simulink model "sampleModel1805"  (R2023a)
settings: Solver=VariableStepAuto  StartTime=0.0  StopTime=10.0  RelTol=1e-3
libraries: hdlsllib x3
settings Model: Creator=user1  LastModifiedBy=user1

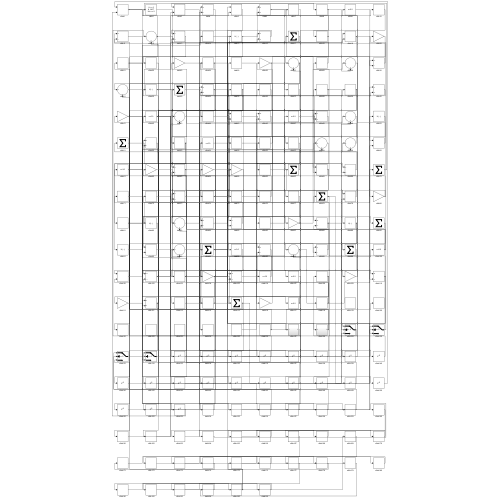
[thumbnail: Simulink's stored preview of the top-level diagram]
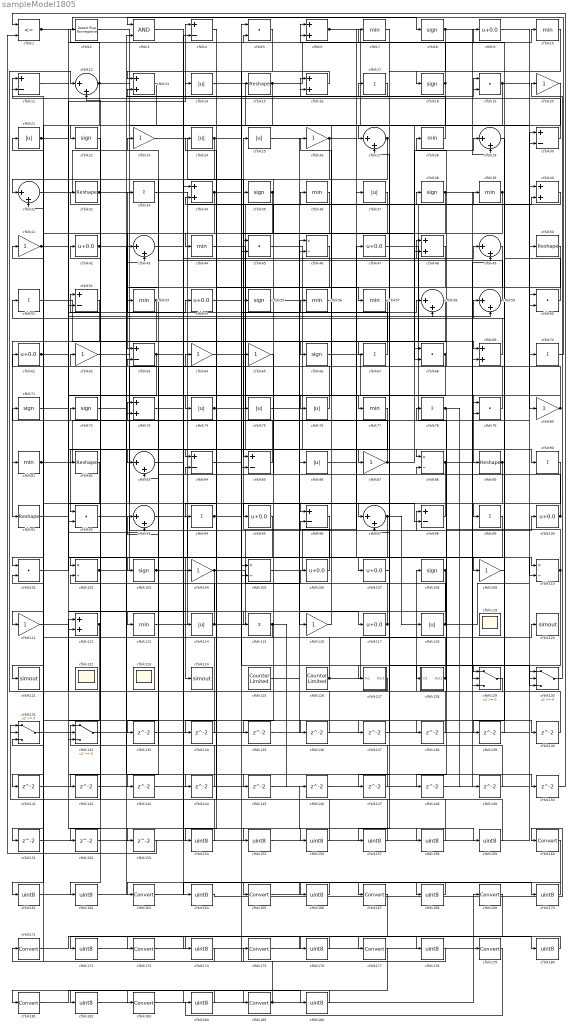
== system sampleModel1805 ==
  cfblk1 : RelationalOperator  Operator=<=  OutDataTypeStr=boolean  InputSameDT=off
  cfblk{7,10,28,36,39,44,53,56..57,77,81,113} (12 alike) : MinMax
  cfblk{9,42,47,54,61,95,100,106..107,117} (10 alike) : Bias  Bias=0.0  SaturateOnIntegerOverflow=off
  cfblk{5,19,45,60,68,79,92,101} (8 alike) : DotProduct  OutDataTypeStr=Inherit: Inherit via internal rule
  cfblk{46,88,102,105,110} (5 alike) : Product  Inputs=*/  RndMeth=Zero  SaturateOnIntegerOverflow=on
  cfblk{8,18,22,35,38,55,66,71..72,103,108} (11 alike) : Signum
  cfblk{20,23,26,41,62,64..65,80,87,104,109,111,116} (13 alike) : Gain
  cfblk{4,11,30,52,63,84..85,96,98} (9 alike) : Sum  Inputs=+-
  cfblk{6,13,16,34,40,48,69,73,112} (9 alike) : Sum
  cfblk{14,21,24..25,37,74..76,86,114,118} (11 alike) : Abs  SaturateOnIntegerOverflow=off
  cfblk{17,33,51,67,70,78,90,94,99,115} (10 alike) : Sum  Inputs=+
  cfblk119 : Scope
      settings: Floating=on
  cfblk{12,27,29,31,43,49,58..59,83,93,97} (11 alike) : Sum  Inputs=|++
  cfblk120 : ToWorkspace  VariableName=simout  SaveFormat=Timeseries  SampleTime=-1
  cfblk121 : ToWorkspace  VariableName=simout  SaveFormat=Timeseries  SampleTime=-1
  cfblk122 : Scope
      settings: Floating=on
  cfblk123 : Scope
      settings: Floating=on
  cfblk124 : ToWorkspace  VariableName=simout  SaveFormat=Timeseries  SampleTime=-1
  cfblk125 : hdlsllib/Sources/Counter Limited  uplimit=7  tsamp=-1
  cfblk126 : hdlsllib/Sources/Counter Limited  uplimit=7  tsamp=-1
  cfblk127 : Subsystem
      settings: LibrarySourceBlock=|
      | hdlsllib/Ports &
      | Subsystems/Subsystem
  cfblk128 : Subsystem
      settings: LibrarySourceBlock=|
      | hdlsllib/Ports &
      | Subsystems/Subsystem
  cfblk{129..132} (4 alike) : Switch  SaturateOnIntegerOverflow=off  InputSameDT=off
  cfblk{133..153} (21 alike) : Delay  SampleTime=1
  cfblk{15,32,50,82,89,91} (6 alike) : Reshape
  cfblk{154..159,161..162,164,166,168,170,172,174,176,178,180,182,184,186} (20 alike) : DataTypeConversion  OutDataTypeStr=uint8  SaturateOnIntegerOverflow=off  RndMeth=Floor
  cfblk{160,163,165,167,169,171,173,175,177,179,181,183,185} (13 alike) : DataTypeConversion  SaturateOnIntegerOverflow=off  RndMeth=Floor
  cfblk2 : hdlsllib/Logic and Bit Operations/Detect Rise Nonnegative  vinit=0  OutDataTypeStr=boolean
  cfblk3 : Logic  AllPortsSameDT=off  OutDataTypeStr=boolean
  wires:
  cfblk98/1 -> cfblk62/1
  cfblk78/1 -> cfblk148/1, cfblk149/1
  cfblk113/1 -> cfblk36/1
  cfblk56/1 -> cfblk31/1
  cfblk110/1 -> cfblk39/1, cfblk129/1, cfblk147/1
  cfblk18/1 -> cfblk27/1, cfblk6/2
  cfblk89/1 -> cfblk99/1, cfblk135/1
  cfblk45/1 -> cfblk90/1
  cfblk64/1 -> cfblk77/1
  cfblk93/1 -> cfblk109/1
  cfblk106/1 -> cfblk25/1
  cfblk32/1 -> cfblk96/1, cfblk7/1
  cfblk92/1 -> cfblk96/2
  cfblk23/1 -> cfblk85/1
  cfblk66/1 -> cfblk89/1
  cfblk115/1 -> cfblk31/2, cfblk146/1
  cfblk105/1 -> cfblk47/1
  cfblk30/1 -> cfblk11/1
  cfblk96/1 -> cfblk124/1
  cfblk74/1 -> cfblk38/1, cfblk127/1(In1)
  cfblk2/1 -> cfblk57/1
  cfblk4/1 -> cfblk74/1
  cfblk127/1(Out1) -> cfblk12/1
  cfblk70/1 -> cfblk3/1
  cfblk52/1 -> cfblk91/1
  cfblk84/1 -> cfblk78/1
  cfblk53/1 -> cfblk81/1, cfblk73/2
  cfblk117/1 -> cfblk56/1, cfblk113/1
  cfblk20/1 -> cfblk76/1
  cfblk132/1 -> cfblk46/1
  cfblk49/1 -> cfblk66/1
  cfblk100/1 -> cfblk35/1, cfblk71/1
  cfblk82/1 -> cfblk111/1
  cfblk44/1 -> cfblk116/1
  cfblk35/1 -> cfblk63/1, cfblk162/1
  cfblk12/1 -> cfblk30/2, cfblk2/1, cfblk151/1
  cfblk34/1 -> cfblk102/1, cfblk48/2
  cfblk125/1 -> cfblk46/2
  cfblk116/1 -> cfblk26/1
  cfblk51/1 -> cfblk86/1
  cfblk19/1 -> cfblk60/1, cfblk45/2
  cfblk37/1 -> cfblk55/1
  cfblk90/1 -> cfblk97/1
  cfblk13/1 -> cfblk22/1
  cfblk8/1 -> cfblk29/2, cfblk157/1
  cfblk67/1 -> cfblk33/1
  cfblk80/1 -> cfblk79/1, cfblk11/2
  cfblk108/1 -> cfblk115/1, cfblk143/1
  cfblk107/1 -> cfblk132/1
  cfblk114/1 -> cfblk100/1, cfblk83/2
  cfblk77/1 -> cfblk92/1
  cfblk14/1 -> cfblk37/1
  cfblk126/1 -> cfblk21/1, cfblk120/1
  cfblk58/1 -> cfblk121/1
  cfblk55/1 -> cfblk69/1
  cfblk76/1 -> cfblk65/1
  cfblk75/1 -> cfblk117/1
  cfblk25/1 -> cfblk67/1
  cfblk27/1 -> cfblk53/1, cfblk44/1
  cfblk15/1 -> cfblk10/1, cfblk52/2
  cfblk16/1 -> cfblk13/1
  cfblk31/1 -> cfblk3/2
  cfblk9/1 -> cfblk80/1
  cfblk103/1 -> cfblk98/1, cfblk16/1
  cfblk39/1 -> cfblk92/2, cfblk142/1
  cfblk85/1 -> cfblk32/1
  cfblk62/1 -> cfblk87/1
  cfblk21/1 -> cfblk75/1, cfblk107/1
  cfblk6/1 -> cfblk68/1, cfblk58/2
  cfblk112/1 -> cfblk72/1, cfblk161/1
  cfblk101/1 -> cfblk54/1
  cfblk86/1 -> cfblk48/1
  cfblk60/1 -> cfblk6/1
  cfblk10/1 -> cfblk18/1
  cfblk130/1 -> cfblk20/1
  cfblk79/1 -> cfblk28/1
  cfblk129/1 -> cfblk108/1
  cfblk17/1 -> cfblk13/2
  cfblk128/1(Out1) -> cfblk52/1, cfblk41/1
  cfblk1/1 -> cfblk8/1, cfblk5/2, cfblk159/1
  cfblk81/1 -> cfblk60/2, cfblk114/1
  cfblk97/1 -> cfblk132/2, cfblk118/1
  cfblk33/1 -> cfblk40/2
  cfblk59/1 -> cfblk23/1
  cfblk48/1 -> cfblk94/1
  cfblk68/1 -> cfblk83/1, cfblk133/1
  cfblk11/1 -> cfblk84/1
  cfblk118/1 -> cfblk12/2, cfblk64/1, cfblk70/1
  cfblk95/1 -> cfblk104/1
  cfblk5/1 -> cfblk85/2
  cfblk102/1 -> cfblk15/1, cfblk19/2
  cfblk38/1 -> cfblk110/1, cfblk141/1
  cfblk57/1 -> cfblk82/1
  cfblk42/1 -> cfblk68/2, cfblk144/1, cfblk145/1
  cfblk28/1 -> cfblk4/1
  cfblk65/1 -> cfblk95/1
  cfblk26/1 -> cfblk45/1, cfblk110/2
  cfblk7/1 -> cfblk97/2
  cfblk61/1 -> cfblk59/2, cfblk14/1
  cfblk104/1 -> cfblk106/1, cfblk132/3, cfblk58/1, cfblk17/1
  cfblk36/1 -> cfblk103/1
  cfblk109/1 -> cfblk9/1
  cfblk46/1 -> cfblk105/2
  cfblk54/1 -> cfblk88/1
  cfblk91/1 -> cfblk98/2
  cfblk69/1 -> cfblk51/1
  cfblk87/1 -> cfblk73/1, cfblk29/1
  cfblk83/1 -> cfblk49/1
  cfblk88/1 -> cfblk130/3, cfblk84/2
  cfblk40/1 -> cfblk34/2
  cfblk41/1 -> cfblk93/2, cfblk140/1
  cfblk24/1 -> cfblk101/1, cfblk19/1
  cfblk63/1 -> cfblk112/2, cfblk136/1
  cfblk94/1 -> cfblk128/1(In1), cfblk129/2, cfblk16/2
  cfblk47/1 -> cfblk69/2
  cfblk133/1 -> cfblk130/2
  cfblk99/1 -> cfblk134/1
  cfblk134/1 -> cfblk34/1
  cfblk135/1 -> cfblk49/2
  cfblk136/1 -> cfblk101/2
  cfblk72/1 -> cfblk137/1
  cfblk137/1 -> cfblk27/2
  cfblk73/1 -> cfblk138/1
  cfblk138/1 -> cfblk112/1
  cfblk29/1 -> cfblk139/1
  cfblk139/1 -> cfblk59/1
  cfblk140/1 -> cfblk88/2
  cfblk141/1 -> cfblk105/1
  cfblk142/1 -> cfblk79/2
  cfblk143/1 -> cfblk130/1
  cfblk144/1 -> cfblk63/2
  cfblk146/1 -> cfblk129/3
  cfblk147/1 -> cfblk93/1
  cfblk148/1 -> cfblk30/1
  cfblk149/1 -> cfblk102/2
  cfblk111/1 -> cfblk150/1
  cfblk150/1 -> cfblk1/1
  cfblk151/1 -> cfblk4/2
  cfblk22/1 -> cfblk152/1
  cfblk152/1 -> cfblk40/1
  cfblk71/1 -> cfblk153/1
  cfblk153/1 -> cfblk1/2
  cfblk50/1 -> cfblk154/1
  cfblk154/1 -> cfblk42/1
  cfblk3/1 -> cfblk155/1
  cfblk155/1 -> cfblk50/1
  cfblk131/1 -> cfblk156/1
  cfblk156/1 -> cfblk24/1
  cfblk157/1 -> cfblk131/1
  cfblk145/1 -> cfblk158/1
  cfblk158/1 -> cfblk131/2
  cfblk159/1 -> cfblk131/3
  cfblk161/1 -> cfblk43/1
  cfblk162/1 -> cfblk43/2
  cfblk43/1 -> cfblk164/1
  cfblk164/1 -> cfblk160/1
  cfblk160/1 -> cfblk166/1
  cfblk166/1 -> cfblk163/1
  cfblk163/1 -> cfblk168/1
  cfblk168/1 -> cfblk165/1
  cfblk165/1 -> cfblk170/1
  cfblk170/1 -> cfblk167/1
  cfblk167/1 -> cfblk172/1
  cfblk172/1 -> cfblk169/1
  cfblk169/1 -> cfblk174/1
  cfblk174/1 -> cfblk171/1
  cfblk171/1 -> cfblk176/1
  cfblk176/1 -> cfblk173/1
  cfblk173/1 -> cfblk178/1
  cfblk178/1 -> cfblk175/1
  cfblk175/1 -> cfblk180/1
  cfblk180/1 -> cfblk177/1
  cfblk177/1 -> cfblk182/1
  cfblk182/1 -> cfblk179/1
  cfblk183/1 -> cfblk185/1
  cfblk179/1 -> cfblk184/1
  cfblk184/1 -> cfblk181/1
  cfblk185/1 -> cfblk5/1, cfblk61/1
  cfblk181/1 -> cfblk186/1
  cfblk186/1 -> cfblk183/1

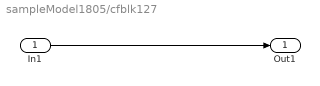
== system sampleModel1805/cfblk127 ==
  In1 : Inport
  Out1 : Outport
  wires:
  In1/1 -> Out1/1

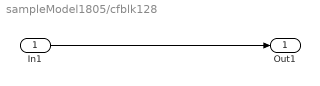
== system sampleModel1805/cfblk128 ==
  In1 : Inport
  Out1 : Outport
  wires:
  In1/1 -> Out1/1
